simulink model "Teach_Pendant_Task_Space"  (Simulink 10.1)
settings: Solver=ode1  StartTime=0.0  StopTime=10  FixedStep=0.001  RelTol=1e-3  EnableMultiTasking=on
values from neighbouring files (symbols this model uses):
  pos = [ ... (first row only)    [get_points.m]
  traj_pos = [pos(1,:); traj_pos]    [MakeLinearTrajectory_TaskSpace.m]
  traj_zone = [1; traj_zone]    [MakeLinearTrajectory_TaskSpace.m]
undefined symbols (not defined in the file or in its folder): qc_get_step_size, starting_point
libraries: quarc_library x3, simulink_need_slupdate x1
settings Model: Creator=RSamra  LastModifiedBy=EE  SimulationMode=external  ExtModeTrigDuration=10100
settings SolverCC: PositivePriorityOrder=on
settings DataIOCC: LimitDataPoints=on  SignalLoggingSaveFormat=ModelDataLogs
settings OptimizationCC: ExpressionDepthLimit=2147483647  InitFltsAndDblsToZero=on
settings DebuggingCC: AlgebraicLoopMsg=error  SolverPrmCheckMsg=warning  FcnCallInpInsideContextMsg=warning  StateNameClashWarn=warning
settings SFSimCC: SimParseCustomCode=off
settings RTWCC: Description=QUARC Win64 Target  SystemTargetFile=quarc_win64.tlc  TemplateMakefile=quarc_default_tmf
settings STFCustomTargetCC: TargetPreCompLibLocation=C:\PROGRA~3\QUARC\lib\2020a\win64\release  ConcurrentExecutionCompliant=on  CombineOutputUpdateFcns=on  CPPClassGenCompliant=on  GRTInterface=off  SystemTargetFile=quarc_win64.tlc
settings GRTTargetCC: TargetPreCompLibLocation=C:\PROGRA~3\QUARC\lib\2020a\win64\release  ParMdlRefBuildCompliant=off  CompOptLevelCompliant=off  CombineOutputUpdateFcns=on  MatFileLogging=off  GRTInterface=off  UseToolchainInfoCompliant=off  ExtMode=on  ExtModeMexFile=quarc_comm

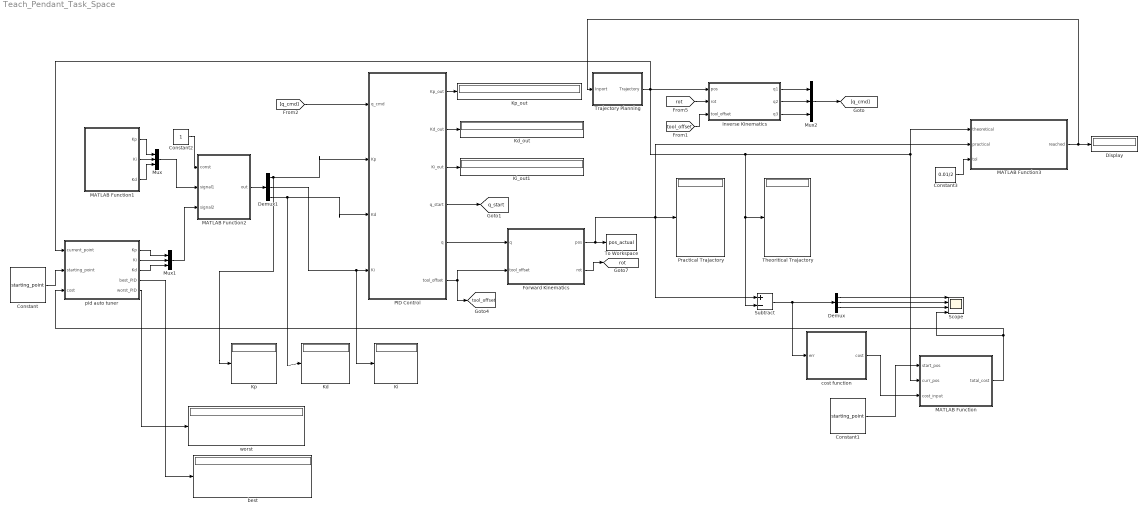
== system Teach_Pendant_Task_Space ==
  Constant : Constant  Value=starting_point
  Constant1 : Constant  Value=starting_point
  Constant2 : Constant
  Constant3 : Constant  Value=0.01/2
  Demux : Demux  Outputs=3
  Demux1 : Demux  Outputs=3
  Display : Display
  Forward Kinematics : MATLAB Function  TreatAsAtomicUnit=on
  Inverse Kinematics : MATLAB Function  TreatAsAtomicUnit=on
  Kd : Display
  Kd_out : Display
      settings: Decimation=100
  Ki : Display
  Ki_out1 : Display
      settings: Decimation=100
  Kp : Display
  Kp_out : Display
      settings: Decimation=100
  MATLAB Function : MATLAB Function  TreatAsAtomicUnit=on
  MATLAB Function1 : MATLAB Function  TreatAsAtomicUnit=on
  MATLAB Function2 : MATLAB Function  TreatAsAtomicUnit=on
  MATLAB Function3 : MATLAB Function  TreatAsAtomicUnit=on
  Mux : Mux  Inputs=3
  Mux1 : Mux  Inputs=3
  Mux2 : Mux  Inputs=3
  PID Control : Subsystem
  Practical Trajactory : Display
  Scope : Scope  NumInputPorts=4
  Subtract : Sum  Inputs=+-
  Theoritical Trajactory : Display
  To Workspace : ToWorkspace  VariableName=pos_actual  SampleTime=-1
  Trajectory Planning : Subsystem
  best : Display
  cost function : MATLAB Function  TreatAsAtomicUnit=on
  pid auto tuner : MATLAB Function  TreatAsAtomicUnit=on
  worst : Display
  tag scope: q_start=global, rot=global, tool_offset=global
  wires:
  PID Control/4(q_start) -> [q_start]
  [q_cmd] -> PID Control/1(q_cmd)
  PID Control/1(Kp_out) -> Kp_out/1
  PID Control/2(Kd_out) -> Kd_out/1
  [tool_offset] -> Inverse Kinematics/3(tool_offset)
  Inverse Kinematics/1(q1) -> Mux2/1
  Inverse Kinematics/2(q2) -> Mux2/2
  Inverse Kinematics/3(q3) -> Mux2/3
  PID Control/6(tool_offset) -> Forward Kinematics/2(tool_offset), [tool_offset]
  Forward Kinematics/1(pos) -> Subtract/1, MATLAB Function3/2(practical), Practical Trajactory/1, To Workspace/1
  Forward Kinematics/2(rot) -> [rot]
  [rot] -> Inverse Kinematics/2(rot)
  PID Control/5(q) -> Forward Kinematics/1(q)
  PID Control/3(Ki_out) -> Ki_out1/1
  Mux2/1 -> [q_cmd]
  Trajectory Planning/1(Trajectory) -> pid auto tuner/1(current_point), MATLAB Function/2(curr_pos), MATLAB Function3/1(theoretical), Subtract/2, Theoritical Trajactory/1, Inverse Kinematics/1(pos)
  Demux/3 -> Scope/3
  Demux/2 -> Scope/2
  Demux/1 -> Scope/1
  Subtract/1 -> cost function/1(err), Demux/1
  Constant/1 -> pid auto tuner/2(starting_point)
  cost function/1(cost) -> MATLAB Function/3(cost_input)
  Constant1/1 -> MATLAB Function/1(start_pos)
  MATLAB Function/1(total_cost) -> pid auto tuner/3(cost), Scope/4
  pid auto tuner/5(worst_PID) -> worst/1
  pid auto tuner/4(best_PID) -> best/1
  MATLAB Function1/1(Kp) -> Mux/1
  MATLAB Function1/2(Ki) -> Mux/2
  MATLAB Function1/3(Kd) -> Mux/3
  MATLAB Function2/1(out) -> Demux1/1
  Demux1/1 -> Kp/1, PID Control/2(Kp)
  Demux1/2 -> Ki/1, PID Control/4(Ki)
  Demux1/3 -> Kd/1, PID Control/3(Kd)
  pid auto tuner/1(Kp) -> Mux1/1
  pid auto tuner/2(Ki) -> Mux1/2
  pid auto tuner/3(Kd) -> Mux1/3
  Mux1/1 -> MATLAB Function2/3(signal2)
  Constant2/1 -> MATLAB Function2/1(const)
  Mux/1 -> MATLAB Function2/2(signal1)
  Constant3/1 -> MATLAB Function3/3(tol)
  MATLAB Function3/1(reached) -> Trajectory Planning/1(Inport), Display/1

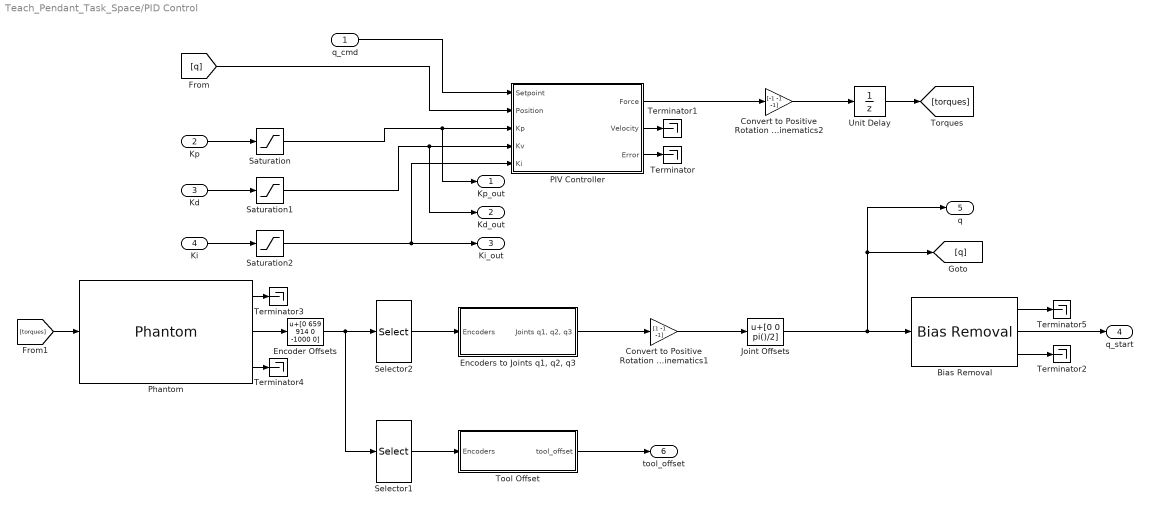
== system Teach_Pendant_Task_Space/PID Control ==
  q_cmd : Inport
  Kp : Inport  Port=2
  Kd : Inport  Port=3
  Ki : Inport  Port=4
  Bias Removal : quarc_library/Discrete/Bias Removal  start_time=0  end_time=qc_get_step_size  switch_id=X  sample_time=qc_get_step_size
      settings: SourceProductName=QUARC Targets
  Convert to Positive Rotation Convension Used in Kinematics1 : Gain  Gain=[1 -1 -1]
  Convert to Positive Rotation Convension Used in Kinematics2 : Gain  Gain=[-1 -1 -1]
  Encoder Offsets : Bias  Bias=[0 659 914 0 -1000 0]
  "Encoders to Joints q1, q2, q3" : Subsystem
  Joint Offsets : Bias  Bias=[0 0 pi()/2]
  PIV Controller : Subsystem
  Phantom : quarc_library/Devices/Third-Party/SensAble/Phantom/Phantom  device_name=Default Device  output_type=Encoders Values  input_type=Joint space  velocity_limit_option=on  velocity_limit=1200  is_7dof=off  sample_time=-1
      settings: AttributesFormatString=(%<device_name>)  SourceProductName=QUARC Targets
  Saturation : Saturate  UpperLimit=[2 2 1]  LowerLimit=[0 0 0]
  Saturation1 : Saturate  UpperLimit=[.1 .1 .025]  LowerLimit=[.02 .02 0]
  Saturation2 : Saturate  UpperLimit=[2 2 3]  LowerLimit=[0 0 0]
  Selector1 : Selector  InputPortWidth=6  IndexOptions=Index vector (dialog)  Indices=[4:6]  OutputSizes=1
  Selector2 : Selector  InputPortWidth=6  IndexOptions=Index vector (dialog)  Indices=[1:3]  OutputSizes=1
  Terminator{,1..5} (6 alike) : Terminator
  Tool Offset : MATLAB Function  TreatAsAtomicUnit=on
  Unit Delay : UnitDelay  SampleTime=-1  HasFrameUpgradeWarning=on
  Kp_out : Outport
  Kd_out : Outport  Port=2
  Ki_out : Outport  Port=3
  q_start : Outport  Port=4
  q : Outport  Port=5
  tool_offset : Outport  Port=6
  wires:
  Saturation2/1 -> Ki_out/1, PIV Controller/5(Ki)
  Ki/1 -> Saturation2/1
  Saturation1/1 -> Kd_out/1, PIV Controller/4(Kv)
  Kd/1 -> Saturation1/1
  Saturation/1 -> Kp_out/1, PIV Controller/3(Kp)
  Kp/1 -> Saturation/1
  "Encoders to Joints q1, q2, q3"/1("Joints q1, q2, q3") -> Convert to Positive Rotation Convension Used in Kinematics1/1
  Selector2/1 -> "Encoders to Joints q1, q2, q3"/1(Encoders)
  Convert to Positive Rotation Convension Used in Kinematics1/1 -> Joint Offsets/1
  q_cmd/1 -> PIV Controller/1(Setpoint)
  PIV Controller/2(Velocity) -> Terminator1/1
  PIV Controller/3(Error) -> Terminator/1
  PIV Controller/1(Force) -> Convert to Positive Rotation Convension Used in Kinematics2/1
  [q] -> PIV Controller/2(Position)
  Phantom/2 -> Encoder Offsets/1
  Phantom/3 -> Terminator4/1
  Phantom/1 -> Terminator3/1
  Encoder Offsets/1 -> Selector2/1, Selector1/1
  Joint Offsets/1 -> Bias Removal/1, q/1, [q]
  Selector1/1 -> Tool Offset/1(Encoders)
  Tool Offset/1(tool_offset) -> tool_offset/1
  Bias Removal/2 -> q_start/1
  [torques] -> Phantom/1
  Convert to Positive Rotation Convension Used in Kinematics2/1 -> Unit Delay/1
  Unit Delay/1 -> [torques]
  Bias Removal/1 -> Terminator5/1
  Bias Removal/3 -> Terminator2/1

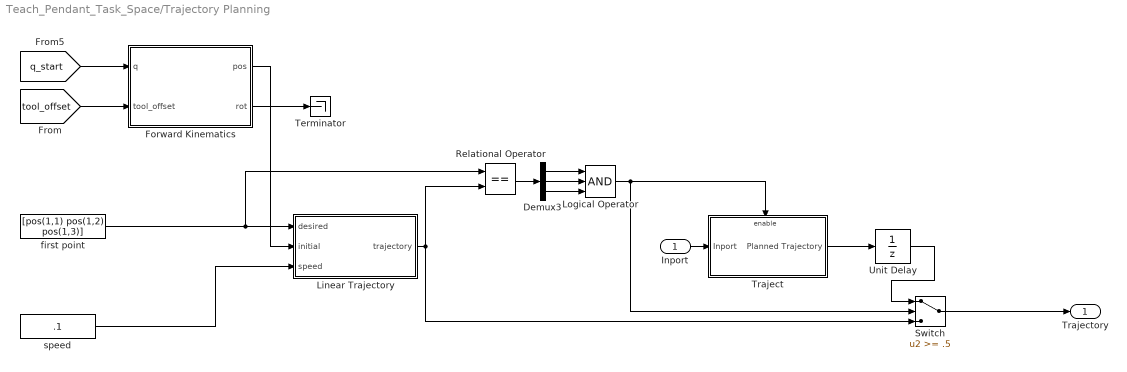
== system Teach_Pendant_Task_Space/Trajectory Planning ==
  Inport : Inport
  Demux3 : Demux  Outputs=3
  Forward Kinematics : MATLAB Function  TreatAsAtomicUnit=on
  Linear Trajectory : Subsystem  Priority=1
  Logical Operator : Logic  Inputs=3  AllPortsSameDT=off  OutDataTypeStr=boolean
  Relational Operator : RelationalOperator  Operator===  OutDataTypeStr=boolean  RndMeth=Nearest
  Switch : Switch  Threshold=.5
  Terminator : Terminator
  Traject : Subsystem
  Unit Delay : UnitDelay  SampleTime=-1  HasFrameUpgradeWarning=on
  first point : Constant  Value=[pos(1,1) pos(1,2) pos(1,3)]
  speed : Constant  Value=.1
  Trajectory : Outport
  wires:
  first point/1 -> Linear Trajectory/1(desired), Relational Operator/1
  Linear Trajectory/1(trajectory) -> Relational Operator/2, Switch/3
  speed/1 -> Linear Trajectory/3(speed)
  Relational Operator/1 -> Demux3/1
  Demux3/1 -> Logical Operator/1
  Demux3/2 -> Logical Operator/2
  Demux3/3 -> Logical Operator/3
  Logical Operator/1 -> Switch/2, Traject/Enable
  Forward Kinematics/1(pos) -> Linear Trajectory/2(initial)
  [tool_offset] -> Forward Kinematics/2(tool_offset)
  [q_start] -> Forward Kinematics/1(q)
  Forward Kinematics/2(rot) -> Terminator/1
  Switch/1 -> Trajectory/1
  Inport/1 -> Traject/1(Inport)
  Traject/1(Planned Trajectory) -> Unit Delay/1
  Unit Delay/1 -> Switch/1

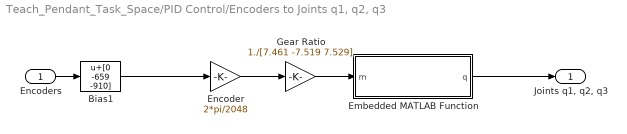
== system Teach_Pendant_Task_Space/PID Control/Encoders to Joints q1, q2, q3 ==
  Encoders : Inport
  Bias1 : Bias  Bias=[0 -659 -910]
  Embedded MATLAB Function : MATLAB Function  TreatAsAtomicUnit=on
  Encoder : Gain  Gain=2*pi/2048
  Gear Ratio : Gain  Gain=1./[7.461 -7.519 7.529]
  "Joints q1, q2, q3" : Outport
  wires:
  Embedded MATLAB Function/1(q) -> "Joints q1, q2, q3"/1
  Encoders/1 -> Bias1/1
  Encoder/1 -> Gear Ratio/1
  Gear Ratio/1 -> Embedded MATLAB Function/1(m)
  Bias1/1 -> Encoder/1

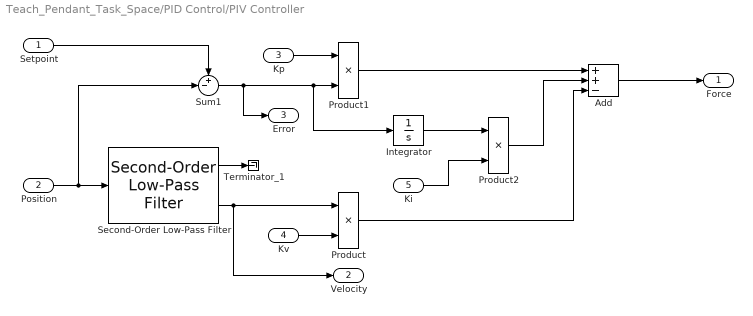
== system Teach_Pendant_Task_Space/PID Control/PIV Controller ==
  Setpoint : Inport
  Position : Inport  Port=2
  Kp : Inport  Port=3
  Kv : Inport  Port=4
  Ki : Inport  Port=5
  Add : Sum  Inputs=++-
  Integrator : Integrator
  Product : Product  RndMeth=Zero
  Product1 : Product  RndMeth=Zero
  Product2 : Product  RndMeth=Zero
  Second-Order Low-Pass Filter : quarc_library/Continuous/Second-Order Low-Pass Filter  params_source=Internal (dialog parameters)  input_width=200  input_zeta=1  input_init=0
  Sum1 : Sum  Inputs=+-|
  Terminator_1 : Terminator
  Force : Outport
  Velocity : Outport  Port=2
  Error : Outport  Port=3
  wires:
  Position/1 -> Sum1/2, Second-Order Low-Pass Filter/1
  Second-Order Low-Pass Filter/2 -> Velocity/1, Product/1
  Kp/1 -> Product1/1
  Setpoint/1 -> Sum1/1
  Sum1/1 -> Error/1, Product1/2, Integrator/1
  Kv/1 -> Product/2
  Second-Order Low-Pass Filter/1 -> Terminator_1/1
  Integrator/1 -> Product2/1
  Ki/1 -> Product2/2
  Product1/1 -> Add/1
  Product2/1 -> Add/2
  Product/1 -> Add/3
  Add/1 -> Force/1

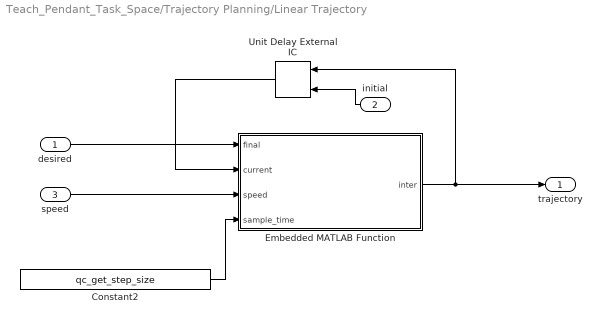
== system Teach_Pendant_Task_Space/Trajectory Planning/Linear Trajectory ==
  desired : Inport
  initial : Inport  Port=2
  speed : Inport  Port=3
  Constant2 : Constant  Value=qc_get_step_size
  Embedded MATLAB Function : MATLAB Function  TreatAsAtomicUnit=on
  Unit Delay External IC : simulink_need_slupdate/Unit Delay External IC  tsamp=-1
      settings: SourceProductBaseCode=SL
  trajectory : Outport
  wires:
  initial/1 -> Unit Delay External IC/2
  speed/1 -> Embedded MATLAB Function/3(speed)
  desired/1 -> Embedded MATLAB Function/1(final)
  Unit Delay External IC/1 -> Embedded MATLAB Function/2(current)
  Constant2/1 -> Embedded MATLAB Function/4(sample_time)
  Embedded MATLAB Function/1(inter) -> trajectory/1, Unit Delay External IC/1

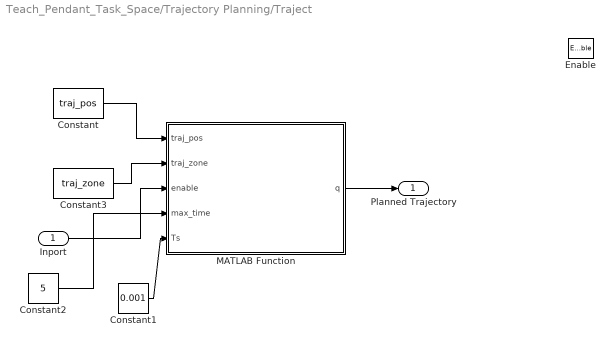
== system Teach_Pendant_Task_Space/Trajectory Planning/Traject ==
  Inport : Inport
  Enable : EnablePort  StatesWhenEnabling=reset
  Constant : Constant  Value=traj_pos
  Constant1 : Constant  Value=0.001
  Constant2 : Constant  Value=5
  Constant3 : Constant  Value=traj_zone
  MATLAB Function : MATLAB Function  TreatAsAtomicUnit=on
  Planned Trajectory : Outport
  wires:
  MATLAB Function/1(q) -> Planned Trajectory/1
  Constant/1 -> MATLAB Function/1(traj_pos)
  Inport/1 -> MATLAB Function/3(enable)
  Constant3/1 -> MATLAB Function/2(traj_zone)
  Constant1/1 -> MATLAB Function/5(Ts)
  Constant2/1 -> MATLAB Function/4(max_time)

== matlab function Trajectory Planning/Forward Kinematics ==
  data: pos output double; q input double; rot output double; tool_offset input double
function [pos,rot]    = ForwardKinematics(q,tool_offset)
% This block supports the Embedded MATLAB subset.
% See the help menu for details. 

% Link lengths
L1 = .132;
L2 = .132;

%Define A-matrices
%A1= DH(theta ,d ,a ,alpha)
A1 = DH(q(1), 0, 0, -pi()/2);
A2 = DH(q(2), 0, L1, 0);
A3 = DH(q(3)-pi/2, 0, L2, 0);

%Define T Matrices
T01=A1;
T02=T01*A2;
T03=T02*A3;

%tool_offset given with respect to frame 3.
T_tool=T03*tool_offset;
rot=T_tool(1:3,1:3);
pos=T_tool(1:3,4);


end

function A = DH(theta, d, a, alpha)

A_R_z = [cos(theta) -sin(theta) 0 0;
         sin(theta) cos(theta) 0 0;
         0 0 1 0;
         0 0 0 1];

A_T_z = [1 0 0 0;
         0 1 0 0;
         0 0 1 d;
         0 0 0 1];
     
  

A_T_x = [1 0 0 a;
         0 1 0 0;
         0 0 1 0;
         0 0 0 1];

A_R_x = [1 0 0 0;
         0 cos(alpha) -sin(alpha)  0;
         0 sin(alpha) cos(alpha) 0;
         0 0 0 1];

A = A_R_z*A_T_z*A_T_x*A_R_x;

end

== matlab function PID Control/Tool Offset ==
  data: Encoders input double; tool_offset output double
function tool_offset = getToolOffset(Encoders)

%convert encoder values to angles using bias and gain
bias = [-2048 -2654 -2048];
gain = [2*pi()/4915 2*pi()/4096 2*pi()/4915];
Angle = (Encoders' + bias).*gain;

% convert the angle to the positive rotation convention defined
% by DH parameters
pos_rot = [-1 1 1];
joint_offset = [0 -(40-180)*pi/180 0];
Joint456 = Angle.*pos_rot + joint_offset;

%pick off theta4 and theta5
theta4 = Joint456(1);
theta5 = Joint456(2);

% The orientation of the tool offset matrix is given two successive
% rotations about x and z axis. 
RotZ = [cos(theta5) -sin(theta5) 0; sin(theta5) cos(theta5) 0; 0 0 1];
RotX = [1 0 0; 0 cos(theta4) -sin(theta4); 0 sin(theta4) cos(theta4)];
R = RotX*RotZ; % R is the rotation matrix of the tool offset matrix with respect to frame 3

% with respect to frame 3, the tool is 0.039m in the x-direction. Convert
% this vector to tool frame coordinates
tool_pos =R * [.039; 0; 0];

%create a Tool_offset transformation matrix. Use Identity matrix for
%rotation to show that the end effector frame and frame 3 are always
%aligned
I = [1 0 0; 0 1 0; 0 0 1];
tool = cat(2,I,tool_pos);
tool_offset = cat(1,tool,[0 0 0 1]);

== matlab function Trajectory Planning/Linear Trajectory/Embedded MATLAB Function ==
  data: final input double; inter output double; current input double; speed input double; sample_time input double
function inter = linear_interpolator( final, current, speed, sample_time)

step = speed*sample_time;
inter = current + sign(final-current).*step;


for i = 1:length(final)
    if ( abs (final(i)-current(i)) < step(i))
        inter(i) = final(i);
    end
end
end

== matlab function cost function ==
  data: err input double; cost output double
function cost = compute_cost_block(err)
% err is a 1x3 or 3x1 vector: [ex ey ez]

% Unpack
ex = err(1);
ey = err(2);
ez = err(3);

% Compute instantaneous cost (squared error)
cost = ex^2 + ey^2 + ez^2;
end

== matlab function pid auto tuner ==
  settings: updateMethod=DISCRETE  sampleTime=0.001
  data: Kp output double; Ki output double; Kd output double; current_point input double; starting_point input double; cost input double; best_PID output double; worst_PID output double
function [Kp, Ki, Kd, best_PID, worst_PID] = pid_auto_tuner(current_point, starting_point, cost)
% Online PSO PID tuner (robust, non-intrusive)
% One particle evaluated per lap; PSO epoch update after all particles are tested.

persistent particles velocities pbest pbest_cost gbest gbest_cost ...
           current_particle initialized in_zone_prev eval_count

% User parameters
NUM_PARTICLES = 10 * 2;   % swarm size
DIM = 6;              % Ki1 Ki2 Ki3 Kd1 Kd2 Kd3 (Kp fixed)
tol = 0.05;           % start-zone radius (meters)
w  = 0.7;             % inertia
c1 = 1.5;             % cognitive weight
c2 = 1.5 * 2;             % social weight

% Initialization
if isempty(initialized)
    particles = rand(NUM_PARTICLES, DIM);     
    velocities = zeros(NUM_PARTICLES, DIM);

    pbest = particles;
    pbest_cost = inf(NUM_PARTICLES,1);

    gbest = particles(1,:);
    gbest_cost = inf;

    current_particle = 1;
    eval_count = 0;
    in_zone_prev = false;

    initialized = true;
end

% Output current particle PIDs
[Kp_vec, Ki_vec, Kd_vec] = scale_and_unpack(particles(current_particle,:));
Kp = Kp_vec(:);
Ki = Ki_vec(:);
Kd = Kd_vec(:);

% Detect start-zone crossing (rising edge)
in_zone = (norm(current_point - starting_point) < tol);
trigger = in_zone && ~in_zone_prev;
in_zone_prev = in_zone;

if trigger

    % 1. Evaluate current particle
    if cost < pbest_cost(current_particle)
        pbest_cost(current_particle) = cost;
        pbest(current_particle,:) = particles(current_particle,:);
    end

    if cost < gbest_cost
        gbest_cost = cost;
        gbest = particles(current_particle,:);
    end

    eval_count = eval_count + 1;

    % 2. Move to next particle
    current_particle = current_particle + 1;
    if current_particle > NUM_PARTICLES
        current_particle = 1;
    end

    % 3. If all particles evaluated, run one PSO epoch update
    if eval_count >= NUM_PARTICLES
        for i = 1:NUM_PARTICLES

            r1 = rand(1, DIM);
            r2 = rand(1, DIM);

            velocities(i,:) = ...
                w  * velocities(i,:) + ...
                c1 .* r1 .* (pbest(i,:) - particles(i,:)) + ...
                c2 .* r2 .* (gbest      - particles(i,:));

            particles(i,:) = particles(i,:) + velocities(i,:);
            particles(i,:) = max(0, min(1, particles(i,:))); % clamp
        end

        eval_count = 0;
    end
end

% Output best PID (global best)
[bKp, bKi, bKd] = scale_and_unpack(gbest);
best_PID = [bKp(:), bKi(:), bKd(:)];

% Output worst PID (highest cost)
[~, worst_idx] = max(pbest_cost);
[wKp, wKi, wKd] = scale_and_unpack(pbest(worst_idx,:));
worst_PID = [wKp(:), wKi(:), wKd(:)];

end


% Helper: scale particle into real PID ranges
function [Kp_vec, Ki_vec, Kd_vec] = scale_and_unpack(x)
% x = [Ki1 Ki2 Ki3 Kd1 Kd2 Kd3] normalized 0..1

Kp_vec = [1.79; 1.46; 0.60];

Ki_vec = zeros(3,1);
Ki_vec(1) = scale(x(1), 0, 2);
Ki_vec(2) = scale(x(2), 0, 2);
Ki_vec(3) = scale(x(3), 0, 3);

Kd_vec = zeros(3,1);
Kd_vec(1) = scale(x(4), 0.02, 0.1);
Kd_vec(2) = scale(x(5), 0.02, 0.1);
Kd_vec(3) = scale(x(6), 0, 0.025);

end

% Helper scaler
function y = scale(val, a, b)
    y = a + val * (b - a);
end

== matlab function MATLAB Function ==
  data: start_pos input double; total_cost output double; curr_pos input double; cost_input input double
function total_cost = cost_sum(start_pos, curr_pos, cost_input)
    persistent cost_sum;

    if isempty(cost_sum)
        cost_sum = 0;
    end

    if all(abs(curr_pos - start_pos) < 1e-6)
        cost_sum = 0;
    else
        cost_sum = cost_sum + cost_input;
    end

    total_cost = cost_sum;
end

== matlab function MATLAB Function1 ==
  data: Kp output double; Ki output double; Kd output double
function [Kp, Ki, Kd] = const_pid()
% Returns constant PID values (no PSO, no auto-tuning)

Kp = [1.79; 1.46; 0.60];
Ki = [1.629; 1.311; 1.316];
Kd = [0.0801; 0.04813; 0.004055];

end

== matlab function PID Control/Encoders to Joints q1, q2, q3/Embedded MATLAB Function ==
  data: m input double; q output double
function q = Motors_2_Joints(m)
q = m;
q(1) = m(1);
q(2) = m(2);
q(3) = m(3) - m(2) -pi/2;
end

== matlab function Forward Kinematics ==
  data: pos output double; q input double; rot output double; tool_offset input double
function [pos,rot]    = ForwardKinematics(q,tool_offset)
% This block supports the Embedded MATLAB subset.
% See the help menu for details. 

% Link lengths
L1 = .132;
L2 = .132;

%Define A-matrices
%A1= DH(theta ,d ,a ,alpha)
A1 = DH(q(1), 0, 0, -pi()/2);
A2 = DH(q(2), 0, L1, 0);
A3 = DH(q(3)-pi/2, 0, L2, 0);

%Define T Matrices
T01=A1;
T02=T01*A2;
T03=T02*A3;

%tool_offset given with respect to frame 3.
T_tool=T03*tool_offset;
rot=T_tool(1:3,1:3);
pos=T_tool(1:3,4);


end

function A = DH(theta, d, a, alpha)

A_R_z = [cos(theta) -sin(theta) 0 0;
         sin(theta) cos(theta) 0 0;
         0 0 1 0;
         0 0 0 1];

A_T_z = [1 0 0 0;
         0 1 0 0;
         0 0 1 d;
         0 0 0 1];
     
  

A_T_x = [1 0 0 a;
         0 1 0 0;
         0 0 1 0;
         0 0 0 1];

A_R_x = [1 0 0 0;
         0 cos(alpha) -sin(alpha)  0;
         0 sin(alpha) cos(alpha) 0;
         0 0 0 1];

A = A_R_z*A_T_z*A_T_x*A_R_x;

end

== matlab function Inverse Kinematics ==
  data: pos input double; rot input double; q1 output double; tool_offset input double; q2 output double; q3 output double
function [q1,q2,q3] = InverseKinematics(pos,rot,tool_offset)
%DESCRIPTION---------------------------------------------------------------
%Compute inverse kinematics using first three joints of OMNI and a tool
%offset.

%INPUTS--------------------------------------------------------------------
%pos - x,y,z position of the tool with respect to the base frame
%rot - Rotation of the tool with respect to the base frame
%tool_offset - x,y,z position and rotation of the tool with respect to frame 3

%OUTPUTS-------------------------------------------------------------------
%q - position of q1, q2, q3

%EXTERNAL REFERENCE--------------------------------------------------------
%Refer to InverseKinematics_from_Geometry.ppt for a diagram of how the inverse kinematics are computed

%Link Lengths
L1 = .132;
L2 = .132;

%Rotate tool_offset from frame 3 to frame 0 coordinates
tool = rot*tool_offset(1:3,4);

% Subtract tool_offset (in frame 0 coord) from the position of the end-effector (in frame 0 coord) 
% to get position of the origin of frame 3.
x = pos(1)-tool(1);
y = pos(2)-tool(2);
z = pos(3)-tool(3);


% distance to frame 3 in x,y plane of base frame
d = sqrt(x^2 + y^2);

%distance to frame 3 in base frame
k = sqrt(d^2+z^2);

% q1 is a function of x and y only
q1 = atan(y/x);

% Using the cosine law: cos(3*pi/2 - q3) = (L1^2+L2^2-k^2)/(2*L1*L2)
q3 = 3*pi/2 - acos((L1^2+L2^2-k^2)/(2*L1*L2));

% phi is positive for z < 0, negative for z > 0, 0 for z = 0.
if (z < 0)
    phi = acos(d/k); 
else
    phi = - acos(d/k);
end

%using the sin law: sin(gamma)/L2 = sin(3*pi/2-q3)/k
gamma = asin((L2*sin(3*pi/2-q3))/k);
q2 = phi-gamma;

== matlab function MATLAB Function2 ==
  data: const input double; out output double; signal1 input double; signal2 input double
function out = select_signal(const, signal1, signal2)
%#codegen

if const == 1
    out = signal1;
else
    out = signal2;
end

end

== matlab function MATLAB Function3 ==
  data: theoretical input double; reached output boolean size=1; practical input double; tol input double
function reached = isWithinTolerance(theoretical, practical, tol)
% theoretical : [3x1] or [1x3]
% practical   : [3x1] or [1x3]
% tol         : scalar
% reached     : true if distance <= tol

% ensure column vectors
theoretical = theoretical(:);
practical   = practical(:);

% Euclidean distance
err = norm(theoretical - practical);

% tolerance check
reached = err <= tol;
end

== matlab function Trajectory Planning/Traject/MATLAB Function ==
  data: q output double; traj_pos input double; traj_zone input double; enable input double; max_time input double; Ts input double
function q = traj_generator(traj_pos, traj_zone, enable, max_time, Ts)

persistent idx N hold_count hold_steps

if isempty(idx)
    idx = 1;
    N = size(traj_pos,1);
    hold_count = 0;
    hold_steps = round(max_time / Ts);
end

q = traj_pos(idx,:)';

is_waypoint = traj_zone(idx) == 1;

if is_waypoint == 1
    
    if enable == 1
        % reached -> advance immediately
        idx = idx + 1;
        if idx > N
            idx = 1;
        end
        hold_count = 0;
        
    else
        % not reached -> wait up to max_time
        if hold_count < hold_steps
            hold_count = hold_count + 1;
        else
            % timeout -> advance anyway
            idx = idx + 1;
            if idx > N
                idx = 1;
            end
            hold_count = 0;
        end
    end
    
else
    % not waypoint -> always advance
    idx = idx + 1;
    if idx > N
        idx = 1;
    end
end
